simulink model "Vienna_Rectifier"  (R2023a)
settings: Solver=ode23t  StartTime=0.0  StopTime=10.0  MaxStep=1e-4  RelTol=1e-3
libraries: spsDiodeLib x6, spsIGBTDiodeLib x6, spsSeriesRLCBranchLib x6, spsVoltageMeasurementLib x3, slpidlib x1, spsThreePhaseVIMeasurementLib x1, spsThreePhaseSourceLib x1, sps_lib x1
settings Model: Creator=Alielden  LastModifiedBy=Alielden

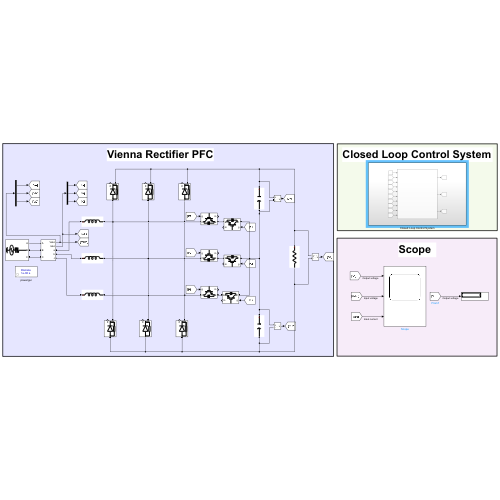
[thumbnail: Simulink's stored preview of the top-level diagram]
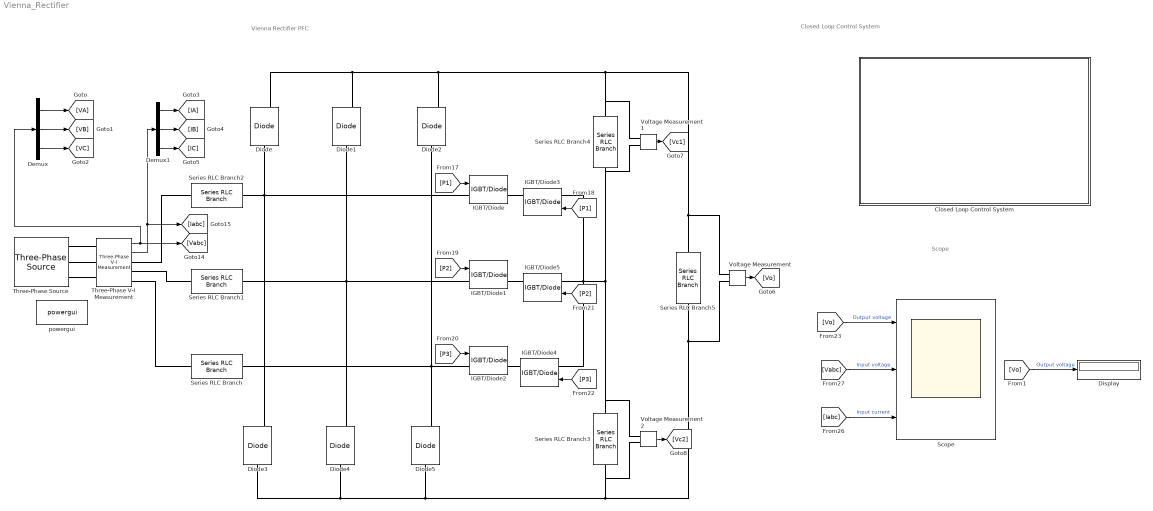
== system Vienna_Rectifier ==
  note: Vienna Rectifier PFC
  note: Closed Loop Control System
  note: Scope
  Closed Loop Control System : Subsystem
  Demux : Demux  Outputs=3
  Demux1 : Demux  Outputs=3
  Diode{,1..5} (6 alike) : spsDiodeLib/Diode  Ron=0.001  Lon=0  Vf=0.8  IC=0  UseSnubber=0  Rs=500  Cs=250e-9  Measurements=on
  Display : Display
  IGBT/Diode{,1..5} (6 alike) : spsIGBTDiodeLib/IGBT//Diode  Ron=1e-3  Rs=1e5  Cs=inf  Measurements=on
  Scope : Scope  NumInputPorts=3
  Series RLC Branch : spsSeriesRLCBranchLib/Series RLC Branch  LConnTagsString=__new0  RConnTagsString=__new0  BranchType=L  Resistance=1  Inductance=1e-3  SetiL0=off  InitialCurrent=0  Capacitance=1e-6  Setx0=off  InitialVoltage=0  Measurements=None
  Series RLC Branch1 : spsSeriesRLCBranchLib/Series RLC Branch  LConnTagsString=__new0  RConnTagsString=__new0  BranchType=L  Resistance=1  Inductance=1e-3  SetiL0=off  InitialCurrent=0  Capacitance=1e-6  Setx0=off  InitialVoltage=0  Measurements=None
  Series RLC Branch2 : spsSeriesRLCBranchLib/Series RLC Branch  LConnTagsString=__new0  RConnTagsString=__new0  BranchType=L  Resistance=1  Inductance=1e-3  SetiL0=off  InitialCurrent=0  Capacitance=1e-6  Setx0=off  InitialVoltage=0  Measurements=None
  Series RLC Branch3 : spsSeriesRLCBranchLib/Series RLC Branch  LConnTagsString=__new0  RConnTagsString=__new0  BranchType=C  Resistance=1  Inductance=1e-3  SetiL0=off  InitialCurrent=0  Capacitance=4000e-6  Setx0=off  InitialVoltage=0  Measurements=None
  Series RLC Branch4 : spsSeriesRLCBranchLib/Series RLC Branch  LConnTagsString=__new0  RConnTagsString=__new0  BranchType=C  Resistance=1  Inductance=1e-3  SetiL0=off  InitialCurrent=0  Capacitance=4000e-6  Setx0=off  InitialVoltage=0  Measurements=None
  Series RLC Branch5 : spsSeriesRLCBranchLib/Series RLC Branch  LConnTagsString=__new0  RConnTagsString=__new0  BranchType=R  Resistance=10  Inductance=1e-3  SetiL0=off  InitialCurrent=0  Capacitance=1e-6  Setx0=off  InitialVoltage=0  Measurements=None
  Three-Phase V-I Measurement : spsThreePhaseVIMeasurementLib/Three-Phase V-I Measurement  VoltageMeasurement=phase-to-ground  SetLabelV=off  LabelV=Vabc  Vpu=off  VpuLL=off  CurrentMeasurement=yes  SetLabelI=off  LabelI=Iabc  Ipu=off  Pbase=100e6  Vbase=500e3  OutputType=Complex  PhasorSimulation=off  PSBequivalent=0
  Three-Phase Source : spsThreePhaseSourceLib/Three-Phase Source  InternalConnection=Yg  VoltagePhases=off  Voltage=380  PhaseAngle=0  Voltage_phases=[25e3 25e3 25e3]/sqrt(3)  PhaseAngles_phases=[0 -120 +120]  Frequency=50  NonIdealSource=on  SpecifyImpedance=off  Resistance=0.000001  Inductance=0  ShortCircuitLevel=100e6  BaseVoltage=25e3  XRratio=7  BusType=swing  Pref=10e3  Qref=0  Prefabc=[10e3, 10e3, 10e3]  Qrefabc=[0, 0, 0]  Qmin=-inf  Qmax=inf
  Voltage Measurement : spsVoltageMeasurementLib/Voltage Measurement  PhasorSimulation=off  OutputType=Complex  PSBequivalent=0
  Voltage Measurement1 : spsVoltageMeasurementLib/Voltage Measurement  PhasorSimulation=off  OutputType=Complex  PSBequivalent=0
  Voltage Measurement2 : spsVoltageMeasurementLib/Voltage Measurement  PhasorSimulation=off  OutputType=Complex  PSBequivalent=0
  powergui : sps_lib/powergui  Priority=1  SimulationMode=Discrete  SampleTime=1e-6  frequency=60  Iterations=50  frequencyindice=50  Pbase=100e6  ErrMax=1e-4  UnitsV=kV  UnitsW=MW  buscounter=0  FunctionMessages=off  echomessages=off  EnableUseOfTLC=off  CurrentSourceSwitches=off  DisableSnubberDevices=off  DisableRonSwitches=off  DisableVfSwitches=off  DisplayEquations=off  AutomaticDiscreteSolvers=off  SolverType=Tustin/Backward Euler (TBE)  Interpol=off  ExternalGateDelay=off  methode=off  Ts=100  x0status=blocks  SPID=on  SwTol=0  HookPort=off  NonlinearTolerance=1e-4  nMaxIteration=100  ContinueOnMaxIteration=off  RestoreLinks=warning  ResistiveCurrentMeasurement=off  Frange=[0:2:500]  Ylog=off  Xlog=on  ShowGrid=off  save=off  variable=ZData  structure=0  ZoomFFT=off  StartTime=0.0  cycles=1  DisplayStyle=1  fundamental=60  FreqAxis=off  MaxFrequency=1000  frequencyindicesteady=1  RmsSteady=1  display=off
  wires:
  Three-Phase V-I Measurement/1 -> [Vabc], Demux/1
  Demux/1 -> [VA]
  Demux/2 -> [VB]
  Demux/3 -> [VC]
  Demux1/1 -> [IA]
  Demux1/2 -> [IB]
  Demux1/3 -> [IC]
  Three-Phase V-I Measurement/2 -> [Iabc], Demux1/1
  Voltage Measurement/1 -> [Vo]
  Voltage Measurement1/1 -> [Vc1]
  Voltage Measurement2/1 -> [Vc2]
  [P1] -> IGBT/Diode/1
  [P1] -> IGBT/Diode3/1
  [P2] -> IGBT/Diode1/1
  [P3] -> IGBT/Diode2/1
  [P2] -> IGBT/Diode5/1
  [P3] -> IGBT/Diode4/1
  [Vo] -> Scope/1  "Output voltage"
  [Vabc] -> Scope/2  "Input voltage"
  [Iabc] -> Scope/3  "Input current"
  [Vo] -> Display/1  "Output voltage"
  connections:
  Three-Phase V-I Measurement/LConn1 -- Three-Phase Source/RConn1
  Three-Phase Source/RConn2 -- Three-Phase V-I Measurement/LConn2
  Three-Phase Source/RConn3 -- Three-Phase V-I Measurement/LConn3
  Three-Phase V-I Measurement/RConn1 -- Series RLC Branch2/LConn1
  Three-Phase V-I Measurement/RConn2 -- Series RLC Branch1/LConn1
  Three-Phase V-I Measurement/RConn3 -- Series RLC Branch/LConn1
  Diode/LConn1 -- IGBT/Diode/LConn1 -- Series RLC Branch2/RConn1 -- Diode3/RConn1
  Diode1/LConn1 -- IGBT/Diode1/LConn1 -- Series RLC Branch1/RConn1 -- Diode4/RConn1
  Diode2/LConn1 -- Series RLC Branch/RConn1 -- IGBT/Diode2/LConn1 -- Diode5/RConn1
  Series RLC Branch5/LConn1 -- Voltage Measurement1/LConn1 -- Series RLC Branch4/LConn1 -- Diode2/RConn1 -- Diode1/RConn1 -- Diode/RConn1 -- Voltage Measurement/LConn1
  Series RLC Branch5/RConn1 -- Voltage Measurement/LConn2 -- Voltage Measurement2/LConn2 -- Series RLC Branch3/RConn1 -- Diode5/LConn1 -- Diode4/LConn1 -- Diode3/LConn1
  IGBT/Diode3/RConn1 -- IGBT/Diode/RConn1
  IGBT/Diode5/RConn1 -- IGBT/Diode1/RConn1
  IGBT/Diode2/RConn1 -- IGBT/Diode4/RConn1
  IGBT/Diode4/LConn1 -- Voltage Measurement2/LConn1 -- Series RLC Branch3/LConn1 -- Voltage Measurement1/LConn2 -- Series RLC Branch4/RConn1 -- IGBT/Diode5/LConn1 -- IGBT/Diode3/LConn1

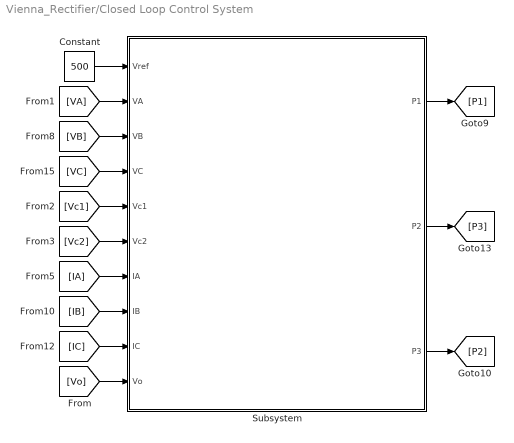
== system Vienna_Rectifier/Closed Loop Control System ==
  Constant : Constant  Value=500
  Subsystem : Subsystem
  wires:
  Subsystem/1(P1) -> [P1]
  Subsystem/3(P3) -> [P2]
  [IA] -> Subsystem/7(IA)
  Constant/1 -> Subsystem/1(Vref)
  [Vo] -> Subsystem/10(Vo)
  [VC] -> Subsystem/4(VC)
  [Vc2] -> Subsystem/6(Vc2)
  [Vc1] -> Subsystem/5(Vc1)
  [VB] -> Subsystem/3(VB)
  [IB] -> Subsystem/8(IB)
  [IC] -> Subsystem/9(IC)
  Subsystem/2(P2) -> [P3]
  [VA] -> Subsystem/2(VA)

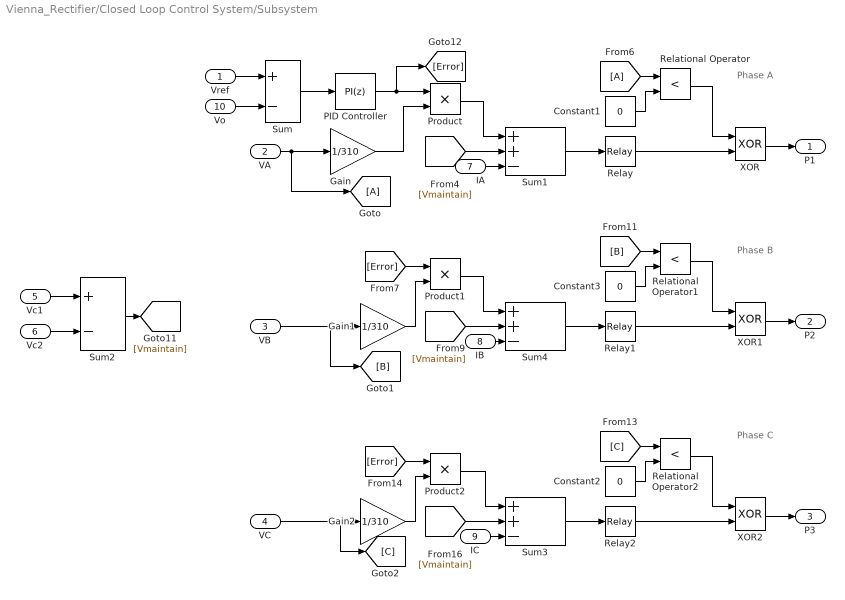
== system Vienna_Rectifier/Closed Loop Control System/Subsystem ==
  note: Phase A
  note: Phase B
  note: Phase C
  Vref : Inport
  VA : Inport  Port=2
  VB : Inport  Port=3
  VC : Inport  Port=4
  Vc1 : Inport  Port=5
  Vc2 : Inport  Port=6
  IA : Inport  Port=7
  IB : Inport  Port=8
  IC : Inport  Port=9
  Vo : Inport  Port=10
  Constant1 : Constant  Value=0
  Constant2 : Constant  Value=0
  Constant3 : Constant  Value=0
  From6 : From
  Gain : Gain  Gain=1/310
  Gain1 : Gain  Gain=1/310
  Gain2 : Gain  Gain=1/310
  Goto : Goto
  PID Controller : slpidlib/PID Controller  Controller=PI  Form=Parallel  TimeDomain=Discrete-time  UseExternalTs=off  SampleTime=1e-6  IntegratorMethod=Forward Euler  FilterMethod=Forward Euler  ControllerParametersSource=internal  P=0.5  I=2500  UseKiTs=off  D=0  N=100  UseFilter=on  TunerSelectOption=Transfer Function Based (PID Tuner App)  InitialConditionSource=internal  InitialConditionForIntegrator=0  InitialConditionForFilter=0  DifferentiatorICPrevScaledInput=0  ExternalReset=none  TrackingMode=off  Kt=1  LimitOutput=on  SatLimitsSource=internal  UpperSaturationLimit=150  LowerSaturationLimit=0  LinearizeAsGain=on  AntiWindupMode=clamping  Kb=1  LimitIntegrator=off  UpperIntegratorSaturationLimit=inf  LowerIntegratorSaturationLimit=-inf  POutMin=[]  POutMax=[]  IOutMin=[]  IOutMax=[]  DOutMin=[]  DOutMax=[]  NOutMin=[]  NOutMax=[]  SumOutMin=[]  SumOutMax=[]  SaturationOutMin=[]  SaturationOutMax=[]  PParamMin=[]  PParamMax=[]  IParamMin=[]  IParamMax=[]  DParamMin=[]  DParamMax=[]  NParamMin=[]  NParamMax=[]  KbParamMin=[]  KbParamMax=[]  KtParamMin=[]  KtParamMax=[]  KbOutMin=[]  KbOutMax=[]  KtOutMin=[]  KtOutMax=[]  IntegratorOutMin=[]  IntegratorOutMax=[]  FilterOutMin=[]  FilterOutMax=[]  SumI1OutMin=[]  SumI1OutMax=[]  SumI2OutMin=[]  SumI2OutMax=[]  SumI3OutMin=[]  SumI3OutMax=[]  SumI4OutMin=[]  SumI4OutMax=[]  SumDOutMin=[]  SumDOutMax=[]  DifferentiatorOutMin=[]  DifferentiatorOutMax=[]  FilterDiffOutCoefMin=[]  FilterDiffOutCoefMax=[]  ReciprocalOutMin=[]  ReciprocalOutMax=[]  SumDenOutMin=[]  SumDenOutMax=[]  SumNumOutMin=[]  SumNumOutMax=[]  DivideOutMin=[]  DivideOutMax=[]  UdiffTsProdOutMin=[]  UdiffTsProdOutMax=[]  NTsProdOutMin=[]  NTsProdOutMax=[]  UintegralTsProdOutMin=[]  UintegralTsProdOutMax=[]  UngainTsProdOutMin=[]  UngainTsProdOutMax=[]  ClampingZeroOutDataTypeStr=Inherit: Inherit via back propagation  ClampingZeroOutMin=[]  ClampingZeroOutMax=[]  FilterDenConstantOutDataTypeStr=Inherit: Inherit via back propagation  FilterDenConstantOutMin=[]  FilterDenConstantOutMax=[]  PCopyOutDataTypeStr=Inherit: Inherit via back propagation  PCopyOutMin=[]  PCopyOutMax=[]  NCopyOutDataTypeStr=Inherit: Inherit via back propagation  NCopyOutMin=[]  NCopyOutMax=[]  IntegratorContinuousStateAttributes=''  IntegratorStateMustResolveToSignalObject=off  IntegratorRTWStateStorageClass=Auto  FilterContinuousStateAttributes=''  FilterStateMustResolveToSignalObject=off  FilterRTWStateStorageClass=Auto  ParallelPVariant=InternalParameters  IdealPVariant=Disabled  IVariant=InternalParameters  DVariant=Disabled  IntegratorVariant=Discrete  SatVariant=Enabled  AWVariant=DiscClampingParallel  PCopyVariant=Disabled  TRVariant=Disabled  FdbkBlocksVariant=Forward  IdealPFdbkVariant=Disabled  SatFdbkVariant=Disabled  DerivativeFilterVariant=Disabled  NVariant=Disabled  NCopyVariant=Disabled_SignalSpec  FilterICVariant=Disabled  IntegratorICVariant=InternalICs  ExternalResetVariant=Disabled  TRSumVariant=Passthrough  SumFdbkVariant=Disabled  SumVariant=Sum_PI  TsampFilterVariant=InternalTs  TsampNgainVariant=Passthrough  TsampIntegralVariant=Disabled_SignalSpec  ExternalSaturationOutDataTypeStr=Inherit: Same as second input
  Product : Product
  Product1 : Product
  Product2 : Product
  Relational Operator : RelationalOperator  Operator=<  OutDataTypeStr=boolean  RndMeth=Simplest  InputSameDT=off
  Relational Operator1 : RelationalOperator  Operator=<  OutDataTypeStr=boolean  RndMeth=Simplest  InputSameDT=off
  Relational Operator2 : RelationalOperator  Operator=<  OutDataTypeStr=boolean  RndMeth=Simplest  InputSameDT=off
  Relay : Relay  OnSwitchValue=1  OffSwitchValue=-1
  Relay1 : Relay  OnSwitchValue=1  OffSwitchValue=-1
  Relay2 : Relay  OnSwitchValue=1  OffSwitchValue=-1
  Sum : Sum  Inputs=+-
  Sum1 : Sum  Inputs=++-
  Sum2 : Sum  Inputs=+-
  Sum3 : Sum  Inputs=++-
  Sum4 : Sum  Inputs=++-
  XOR : Logic  Operator=XOR  AllPortsSameDT=off  OutDataTypeStr=boolean
  XOR1 : Logic  Operator=XOR  AllPortsSameDT=off  OutDataTypeStr=boolean
  XOR2 : Logic  Operator=XOR  AllPortsSameDT=off  OutDataTypeStr=boolean
  P1 : Outport
  P2 : Outport  Port=2
  P3 : Outport  Port=3
  wires:
  Product/1 -> Sum1/1
  Constant3/1 -> Relational Operator1/2
  PID Controller/1 -> [Error], Product/1
  Sum1/1 -> Relay/1
  [Error] -> Product2/1
  Product1/1 -> Sum4/1
  [Vmaintain] -> Sum4/2
  Relational Operator1/1 -> XOR1/1
  Constant1/1 -> Relational Operator/2
  [Error] -> Product1/1
  [Vmaintain] -> Sum1/2
  Relay1/1 -> XOR1/2
  Relay2/1 -> XOR2/2
  Sum2/1 -> [Vmaintain]
  Relational Operator/1 -> XOR/1
  Product2/1 -> Sum3/1
  Gain/1 -> Product/2
  Gain1/1 -> Product1/2
  Constant2/1 -> Relational Operator2/2
  Relational Operator2/1 -> XOR2/1
  Relay/1 -> XOR/2
  [Vmaintain] -> Sum3/2
  Gain2/1 -> Product2/2
  Sum4/1 -> Relay1/1
  Sum3/1 -> Relay2/1
  VB/1 -> [B], Gain1/1
  VC/1 -> [C], Gain2/1
  Vc1/1 -> Sum2/1
  Vc2/1 -> Sum2/2
  IA/1 -> Sum1/3
  IB/1 -> Sum4/3
  IC/1 -> Sum3/3
  VA/1 -> Goto/1, Gain/1
  From6/1 -> Relational Operator/1
  [C] -> Relational Operator2/1
  [B] -> Relational Operator1/1
  Vref/1 -> Sum/1
  Vo/1 -> Sum/2
  Sum/1 -> PID Controller/1
  XOR1/1 -> P2/1
  XOR2/1 -> P3/1
  XOR/1 -> P1/1
